simulink model "simple_mode"  (R2018b)
settings: Solver=VariableStepAuto  StartTime=0.0  StopTime=10.0  RelTol=1e-3
settings Model: Creator=Administrator  LastModifiedBy=Administrator

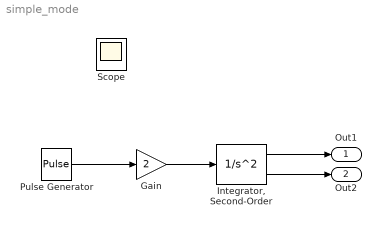
== system simple_mode ==
  Gain : Gain  Gain=2
  "Integrator, Second-Order" : SecondOrderIntegrator
  Pulse Generator : DiscretePulseGenerator  PulseType=Time based  Period=10  PulseWidth=5
  Out1 : Outport
  Out2 : Outport  Port=2
  Scope : Scope
  wires:
  Pulse Generator/1 -> Gain/1
  Gain/1 -> "Integrator, Second-Order"/1
  "Integrator, Second-Order"/1 -> Out1/1
  "Integrator, Second-Order"/2 -> Out2/1
